simulink model "SolverDyn_TestBed"  (R2019b)
settings: Solver=FixedStepDiscrete  StartTime=0.0  StopTime=1  FixedStep=0.01  RelTol=1e-3  EnableMultiTasking=on
undefined symbols (not defined in the file): MWS
libraries: Lib_Solve_IterNRSolverJC_TMATS x1
settings Model: Creator=jwchapm2  LastModifiedBy=bhisma
settings DataIOCC: LimitDataPoints=on  SaveFormat=Array  ReturnWorkspaceOutputs=off
settings OptimizationCC: ExpressionDepthLimit=2147483647  LifeSpan=inf
settings DebuggingCC: UnderspecifiedInitializationDetection=Classic  MergeDetectMultiDrivingBlocksExec=none  SolverPrmCheckMsg=warning  StateNameClashWarn=warning  SFUnexpectedBacktrackingDiag=warning  SFNoUnconditionalDefaultTransitionDiag=warning  SFExecutionAtInitializationDiag=none  ArithmeticOperatorsInVariantConditions=warning
settings HardwareCC: ProdBitPerPointer=32  ProdBitPerSizeT=32  ProdBitPerPtrDiffT=32  ProdLargestAtomicFloat=None  ProdIntDivRoundTo=Undefined  ProdEndianess=Unspecified  ProdWordSize=32  ProdHWDeviceType=32-bit Generic
settings ModelReferenceCC: PropagateSignalLabelsOutOfModel=off
settings SFSimCC: SimUseLocalCustomCode=off  CustomCodeUndefinedFunction=UseInterfaceOnly
settings RTWCC: RTWUseLocalCustomCode=off
settings CodeAppCC: StateflowObjectComments=on
settings GRTTargetCC: TargetLangStandard=C89/C90 (ANSI)  GeneratePreprocessorConditionals=Disable all
settings ConfigComp: CovMetricSettings=dw  CovHtmlReporting=on  CovSaveCumulativeToWorkspaceVar=on  CovSaveSingleToWorkspaceVar=on  CovExternalEMLEnable=off

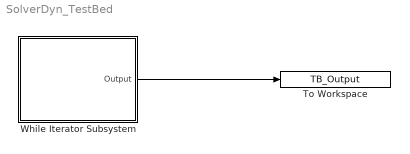
== system SolverDyn_TestBed ==
  To Workspace : ToWorkspace  VariableName=TB_Output  SampleTime=-1
  While Iterator Subsystem : Subsystem  TreatAsAtomicUnit=on
  wires:
  While Iterator Subsystem/1(Output) -> To Workspace/1

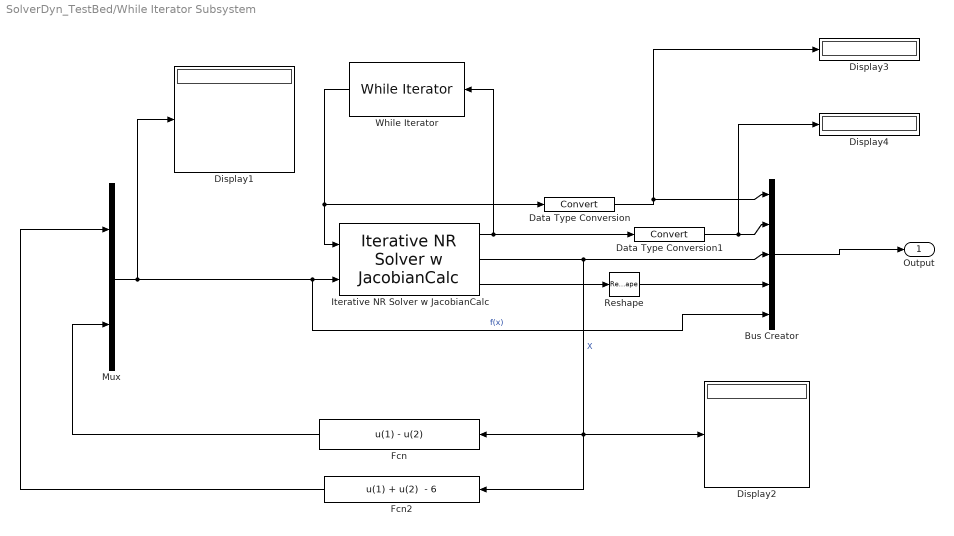
== system SolverDyn_TestBed/While Iterator Subsystem ==
  Bus Creator : BusCreator  Inputs=5
  Data Type Conversion : DataTypeConversion
  Data Type Conversion1 : DataTypeConversion
  Display{1..4} (4 alike) : Display
  Fcn : Fcn  Expr=u(1) - u(2)
  Fcn2 : Fcn  Expr="u(1) + u(2)  - 6"
  Iterative NR Solver w JacobianCalc : Lib_Solve_IterNRSolverJC_TMATS/Iterative NR Solver w JacobianCalc  SJac_Per_M=MWS.SolverDyn.Per  SNR_IC_M=MWS.SolverDyn.IC  SNR_DX_M=MWS.SolverDyn.dX  SJacobianAttempts_M=MWS.SolverDyn.Jatm  Cond_Limits_M=MWS.SolverDyn.Cond_Lim
  Mux : Mux  Inputs=2
  Reshape : Reshape
  While Iterator : WhileIterator  MaxIters=MWS.SolverDyn.Jatm *2  WhileBlockType=do-while  ShowIterationPort=on
  Output : Outport
  wires:
  Mux/1 -> Bus Creator/5, Iterative NR Solver w JacobianCalc/2, Display1/1  "f(x)"
  Iterative NR Solver w JacobianCalc/2 -> Display2/1, Fcn2/1, Fcn/1, Bus Creator/3  "X"
  Fcn/1 -> Mux/2
  Fcn2/1 -> Mux/1
  Bus Creator/1 -> Output/1
  Iterative NR Solver w JacobianCalc/1 -> Data Type Conversion1/1, While Iterator/1
  While Iterator/1 -> Iterative NR Solver w JacobianCalc/1, Data Type Conversion/1
  Data Type Conversion/1 -> Display3/1, Bus Creator/1
  Data Type Conversion1/1 -> Display4/1, Bus Creator/2
  Iterative NR Solver w JacobianCalc/3 -> Reshape/1
  Reshape/1 -> Bus Creator/4
